simulink model "Ejercicio11"  (R2013a)
settings: Solver=ode45  StartTime=0.0  StopTime=10.0  RelTol=1e-3
values from neighbouring files (symbols this model uses):
  a = [-1 0;1 -2]    [ejercicio11.m]
  b = [1 0;0 1]    [ejercicio11.m]
  c = [-1 1]    [ejercicio11.m]
  k = place(a,b,pd)    [ejercicio11.m]
settings Model: Creator=mario  LastModifiedBy=mario

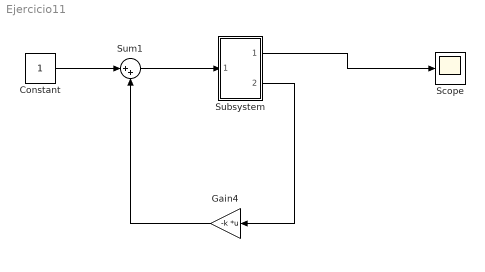
== system Ejercicio11 ==
  Constant : Constant
  Gain4 : Gain  Gain=-k  Multiplication=Matrix(K*u) (u vector)
  Scope : Scope
  Subsystem : Subsystem
  Sum1 : Sum  Inputs=|++
  wires:
  Gain4/1 -> Sum1/2
  Constant/1 -> Sum1/1
  Subsystem/1(Out1) -> Scope/1
  Sum1/1 -> Subsystem/1(In1)
  Subsystem/2(Out2) -> Gain4/1

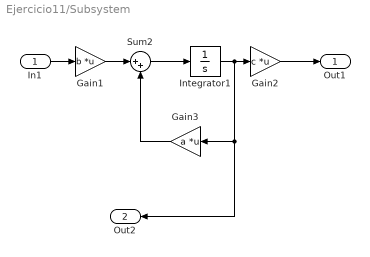
== system Ejercicio11/Subsystem ==
  In1 : Inport
  Gain1 : Gain  Gain=b  Multiplication=Matrix(K*u) (u vector)
  Gain2 : Gain  Gain=c  Multiplication=Matrix(K*u) (u vector)
  Gain3 : Gain  Gain=a  Multiplication=Matrix(K*u) (u vector)
  Integrator1 : Integrator
  Sum2 : Sum  Inputs=|++
  Out1 : Outport
  Out2 : Outport  Port=2
  wires:
  Integrator1/1 -> Out2/1, Gain3/1, Gain2/1
  In1/1 -> Gain1/1
  Gain1/1 -> Sum2/1
  Gain3/1 -> Sum2/2
  Gain2/1 -> Out1/1
  Sum2/1 -> Integrator1/1
